simulink model "vrmanipul"  (Simulink 7.5)
settings: Solver=ode45  StartTime=0.0  StopTime=Inf  RelTol=1e-3
libraries: vrlib x11
Description:
  | Manipulator with Space Mouse
  | 
  | This example illustrates the use of Simulink(R) 3D Animation(TM) for virtual reality prototyping
  | and testing the viability of designs before the implementation phase. Also, this example
  | illustrates the use of the Space Mouse for manipulating objects in a virtual world.
  | 
  | <<html/manipul.gif>>
  | 
  | The VRML model represents a nuclear hot chamber manipulator. It is manipulated
  | by a simple Simulink(R) model containing the Space Mouse Input block.
  | This model uses all 6 degrees of freedom of the Space Mouse for manipulating
  | the mechanic arm, and mouse button 1 to close the grip of manipulator jaws.
  | 
  | Space Mouse is an input device with 6 degrees of freedom.
  | It is useful for navigating and manipulating objects in a virtual world.
  | Space Mouse is also suitable as a general input device for Simulink models.
  | This professional 3-D device greatly facilitates all the above mentioned tasks,
  | and we recommend you use it for higher performance applications and user comfort.
  | Space Mouse is supported through the Space Mouse Input block which is included
  | in the Simulink 3D Animation block library.
  | 
  | The Space Mouse Input block can operate in three modes to cover the most
  | typical use of such a device in 3-D context:
  | 
  |     * Speeds
  |     * Positions
  |     * Viewpoint coordinates
  | 
  | Note: This demo requires the Space Mouse or compatible device (SpaceMouse Plus, SpaceTraveller, PuckMan).
settings Model: Creator=Houska  LastModifiedBy=Houska  CovMetricSettings=d  ExtModeTrigMode=oneshot  ExtModeArmWhenConnect=off
settings DataIOCC: SaveOutput=off  SaveTime=off  SignalLoggingName=logsOut
settings OptimizationCC: BlockReduction=off  BooleanDataType=off  InlineInvariantSignals=on  InitFltsAndDblsToZero=on
settings DebuggingCC: CheckExecutionContextPreStartOutputMsg=on  CheckExecutionContextRuntimeOutputMsg=on  SignalResolutionControl=TryResolveAllWithWarning  SolverPrmCheckMsg=none  MultiTaskDSMMsg=warning  MultiTaskCondExecSysMsg=none  StrictBusMsg=None
settings HardwareCC: TargetUnknown=on
settings ModelReferenceCC: UpdateModelReferenceTargets=IfOutOfDate
settings RTWCC: IncludeERTFirstTime=on
settings GRTTargetCC: TargetFcnLib=ansi_tfl_tmw_new.mat

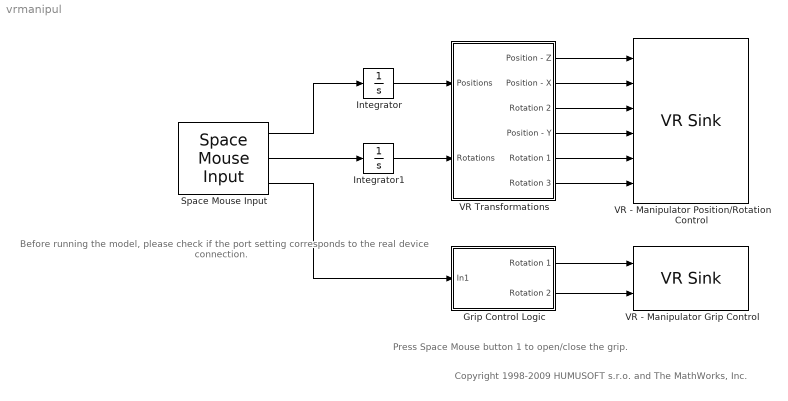
== system vrmanipul ==
  note: Press Space Mouse
      | button 1 to open/close the grip.
  note: Before running the model,
      | please check if the port setting
      | corresponds to the real
      | device connection.
  note: Copyright 1998-2009 HUMUSOFT s.r.o. and The MathWorks, Inc.
  Grip Control Logic : Subsystem
  Integrator : Integrator  InitialCondition=[0 -3 0]  LimitOutput=on  UpperSaturationLimit=[4 1 4]  LowerSaturationLimit=[-4 -4 -4]  ZeroCross=off
  Integrator1 : Integrator  InitialCondition=[0 2 0]  UpperSaturationLimit=Inf  LowerSaturationLimit=-Inf  ZeroCross=off
  Space Mouse Input : vrlib/Space Mouse Input  Port=USB1  OutputType=Speed  Dominant=on  DisableTranslation=off  DisableRotation=off  NormalizeAngle=off  EnableLimit=off  PositionSensitivity=0.001  RotationSensitivity=0.001  InitialPosition=[0 0 0]  InitialRotation=[0 0 0]  PositionLow=[-100 -100 -100]  PositionUp=[100 100 100]
  VR - Manipulator Grip Control : vrlib/VR Sink  InstantiateOnLoad=on  SampleTime=0.2  ViewEnable=on  RemoteChange=off  RemoteView=off  FieldsWritten=Finger1.rotation.4.1.1.double#Finger2.rotation.4.1.1.double  WorldFileName=vrmanipul.wrl  WorldDescription=VR Manipulator  AutoView=off  VideoDimensions=[]
  VR - Manipulator Position/Rotation Control : vrlib/VR Sink  InstantiateOnLoad=on  SampleTime=0.2  ViewEnable=on  RemoteChange=off  RemoteView=off  FieldsWritten=Portal.translation.3.1.1.double#Base.translation.3.1.1.double#Telescope.rotation.4.1.1.double#Telescope.translation.3.1.1.double#Arm.rotation.4.1.1.double#Wrist.rotation.4.1.1.double  WorldFileName=vrmanipul.wrl  WorldDescription=VR Manipulator  AutoView=on  VideoDimensions=[]  FigureProperties="{'Position', 'Name', 'Viewpoint', 'CameraBound', 'CameraDirection', 'CameraPosition', 'CameraUpVector', 'ZoomFactor', 'Antialiasing', 'Headlight', 'Lighting', 'NavPanel', 'StatusBar', 'ToolBar', 'Textures', 'Transparency', 'Wireframe', 'NavZones', 'NavMode', 'NavSpeed', 'Record2DCompressMethod', 'Record2DCompressQuality', 'Record2D', 'Record2DFileName', 'Record2DFPS'; [5.0000000000000000e+000  9.2000000000000000e+001  5.7600000000000000e+002  3.8000000000000000e+002], 'VR Manipulator', 'View1', 'on', [0.0000000000000000e+000  0.0000000000000000e+000 -1.0000000000000000e+000], [0.0000000000000000e+000  0.0000000000000000e+000  0.0000000000000000e+000], [0.0000000000000000e+000  1.0000000000000000e+000  0.0000000000000000e+000], [1.0000000000000000e+000], 'off', 'on', 'on', 'halfbar', 'on', 'on', 'on', 'on', 'off', 'off', 'examine', 'normal', 'auto', [7.5000000000000000e+001], 'off', '%f_anim_%n.avi', [1.5000000000000000e+001]}"
  VR Transformations : Subsystem
  wires:
  Space Mouse Input/3 -> Grip Control Logic/1(In1)
  Space Mouse Input/1 -> Integrator/1
  Integrator/1 -> VR Transformations/1(Positions)
  Space Mouse Input/2 -> Integrator1/1
  Integrator1/1 -> VR Transformations/2(Rotations)
  VR Transformations/1(Position - Z) -> VR - Manipulator Position/Rotation Control/1
  VR Transformations/2(Position - X) -> VR - Manipulator Position/Rotation Control/2
  VR Transformations/3(Rotation 2) -> VR - Manipulator Position/Rotation Control/3
  VR Transformations/4(Position - Y) -> VR - Manipulator Position/Rotation Control/4
  VR Transformations/5(Rotation 1) -> VR - Manipulator Position/Rotation Control/5
  VR Transformations/6(Rotation 3) -> VR - Manipulator Position/Rotation Control/6
  Grip Control Logic/1(Rotation 1) -> VR - Manipulator Grip Control/1
  Grip Control Logic/2(Rotation 2) -> VR - Manipulator Grip Control/2

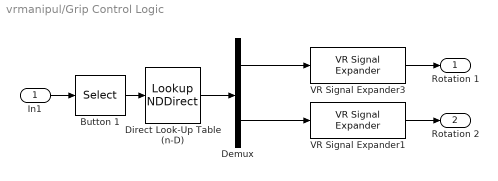
== system vrmanipul/Grip Control Logic ==
  In1 : Inport  OutDataType=sfix(16)  OutScaling=2^0
  Button 1 : Selector  IndexOptions=Index vector (dialog)  Indices=1  OutputSizes=1
  Demux : Demux  Outputs=2
  Direct Look-Up Table (n-D) : LookupNDDirect  InputsSelectThisObjectFromTable=Column  Table=[0.3 0.02;-0.3 -0.02]
  VR Signal Expander1 : vrlib/VR Signal Expander  SystemSampleTime=-1  outwidth=4  outidx=4
  VR Signal Expander3 : vrlib/VR Signal Expander  SystemSampleTime=-1  outwidth=4  outidx=4
  Rotation 1 : Outport  OutDataType=sfix(16)  OutScaling=2^0
  Rotation 2 : Outport  Port=2  OutDataType=sfix(16)  OutScaling=2^0
  wires:
  Button 1/1 -> Direct Look-Up Table (n-D)/1
  Direct Look-Up Table (n-D)/1 -> Demux/1
  Demux/1 -> VR Signal Expander3/1
  Demux/2 -> VR Signal Expander1/1
  VR Signal Expander3/1 -> Rotation 1/1
  In1/1 -> Button 1/1
  VR Signal Expander1/1 -> Rotation 2/1

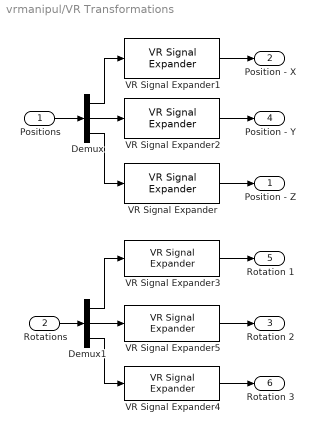
== system vrmanipul/VR Transformations ==
  Positions : Inport  OutDataType=sfix(16)  OutScaling=2^0
  Rotations : Inport  Port=2  OutDataType=sfix(16)  OutScaling=2^0
  Demux : Demux  Outputs=3
  Demux1 : Demux  Outputs=3
  VR Signal Expander : vrlib/VR Signal Expander  SystemSampleTime=-1  outwidth=3  outidx=3
  VR Signal Expander1 : vrlib/VR Signal Expander  SystemSampleTime=-1  outwidth=3  outidx=1
  VR Signal Expander2 : vrlib/VR Signal Expander  SystemSampleTime=-1  outwidth=3  outidx=2
  VR Signal Expander3 : vrlib/VR Signal Expander  SystemSampleTime=-1  outwidth=4  outidx=4
  VR Signal Expander4 : vrlib/VR Signal Expander  SystemSampleTime=-1  outwidth=4  outidx=4
  VR Signal Expander5 : vrlib/VR Signal Expander  SystemSampleTime=-1  outwidth=4  outidx=4
  Position - Z : Outport  OutDataType=sfix(16)  OutScaling=2^0
  Position - X : Outport  Port=2  OutDataType=sfix(16)  OutScaling=2^0
  Rotation 2 : Outport  Port=3  OutDataType=sfix(16)  OutScaling=2^0
  Position - Y : Outport  Port=4  OutDataType=sfix(16)  OutScaling=2^0
  Rotation 1 : Outport  Port=5  OutDataType=sfix(16)  OutScaling=2^0
  Rotation 3 : Outport  Port=6  OutDataType=sfix(16)  OutScaling=2^0
  wires:
  Positions/1 -> Demux/1
  Rotations/1 -> Demux1/1
  VR Signal Expander/1 -> Position - Z/1
  VR Signal Expander1/1 -> Position - X/1
  VR Signal Expander2/1 -> Position - Y/1
  VR Signal Expander3/1 -> Rotation 1/1
  Demux1/1 -> VR Signal Expander3/1
  VR Signal Expander4/1 -> Rotation 3/1
  VR Signal Expander5/1 -> Rotation 2/1
  Demux1/2 -> VR Signal Expander5/1
  Demux1/3 -> VR Signal Expander4/1
  Demux/1 -> VR Signal Expander1/1
  Demux/2 -> VR Signal Expander2/1
  Demux/3 -> VR Signal Expander/1
